simulink model "Shin_com"  (R2024a)
settings: Solver=VariableStepAuto  StartTime=0.0  StopTime=10.0  RelTol=1e-3
undefined symbols (not defined in the file): route1_waypoint_x, route1_waypoint_y, route2_waypoint_x, route2_waypoint_y, route3_waypoint_x, route3_waypoint_y, route4_waypoint_x, route4_waypoint_y, route5_waypoint_x, route5_waypoint_y
libraries: CarMaker4SL x162, slpidlib x4, robotalgslib x1, matrix_library x1
(part 2 of 4)

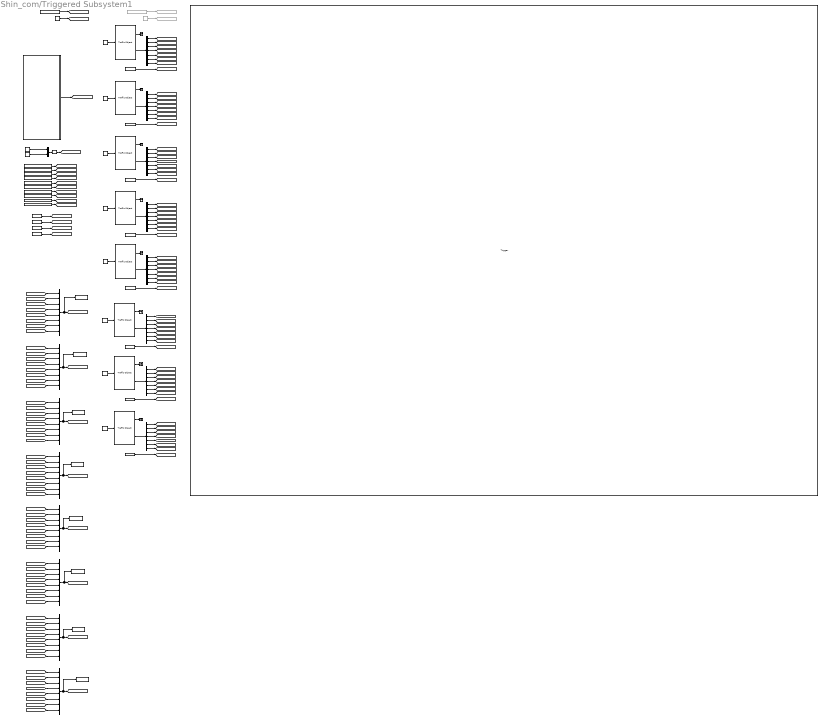
== system Shin_com/Triggered Subsystem1 ==
  note: Traffic Size
      | Length: 4.47
      | Width: 1.97
      | Height: 1.12
  note: Do Not Modify !!
  note: Traffic Size
      | Length: 4.47
      | Width: 1.97
      | Height: 1.12
  note: Traffic Size
      | Length: 4.47
      | Width: 1.97
      | Height: 1.12
  note: Traffic Size
      | Length: 4.47
      | Width: 1.97
      | Height: 1.12
  note: Do Not Modify !!
  note: Traffic Size
      | Length: 4.47
      | Width: 1.97
      | Height: 1.12
  note: Traffic Size
      | Length: 4.47
      | Width: 1.97
      | Height: 1.12
  note: Traffic Size
      | Length: 4.47
      | Width: 1.97
      | Height: 1.12
  note: Traffic Size
      | Length: 4.47
      | Width: 1.97
      | Height: 1.12
  Trigger : TriggerPort  TriggerType=function-call  VariantControl=(inherit)
      mask Display: image('KakaoTalk_20250521_163600732.jpg');
  Bus Selector{3..10} (8 alike) : BusSelector  OutputSignals=t_0 x,t_0 y,v_0 x,v_0 y,a_0 x,a_0 y,r_zyx z
  Constant11 : Constant  Value=28
  Constant12 : Constant  Value=route1_waypoint_y.Data
  Constant13 : Constant  Value=route2_waypoint_y.Data
  Constant14 : Constant  Value=route2_waypoint_x.Data
  Constant15 : Constant  Value=route1_waypoint_x.Data
  Constant16 : Constant  Value=route3_waypoint_y.Data
  Constant17 : Constant  Value=route3_waypoint_x.Data
  Constant18 : Constant  Value=route4_waypoint_y.Data
  Constant19 : Constant  Value=route4_waypoint_x.Data
  Constant20 : Constant  Value=route5_waypoint_y.Data
  Constant21 : Constant  Value=route5_waypoint_x.Data
  Constant22 : Constant  Value=23
  Constant23 : Constant  Value=10/3.6
  Constant25 : Constant  Value=11.5
  Constant26 : Constant  Value=24
  Constant27 : Constant  Value=25
  Constant28 : Constant  Value=26
  Constant29 : Constant  Value=27
  Constant6 : Constant  Commented=on  Value=20/3.6
  Constant7 : Constant  Value=21
  Constant8 : Constant  Value=2.48
  Constant9 : Constant  Value=22
  Goto31 : Goto  Commented=on  GotoTag=CrossTrackError
  Goto64 : Goto  Commented=on  GotoTag=Target_Speed
  Mux{,1..2,5..9} (8 alike) : Mux  Inputs=8
  Mux4 : Mux  Inputs=2
  Read CM Dict10 : CarMaker4SL/Read CM Dict  xname=Car.Fr1.tx  xsync=off  xstime=Inherited
  Read CM Dict11 : CarMaker4SL/Read CM Dict  xname=Car.Fr1.ty  xsync=off  xstime=Inherited
  Read CM Dict12 : CarMaker4SL/Read CM Dict  xname=Car.Fr1.rz  xsync=off  xstime=Inherited
  Read CM Dict13 : CarMaker4SL/Read CM Dict  xname=Car.v  xsync=off  xstime=Inherited
  Read CM Dict14 : CarMaker4SL/Read CM Dict  xname=Traffic.T24.rzv  xsync=off  xstime=Inherited
  Read CM Dict15 : CarMaker4SL/Read CM Dict  xname=Traffic.T25.rzv  xsync=off  xstime=Inherited
  Read CM Dict16 : CarMaker4SL/Read CM Dict  xname=Traffic.T26.rzv  xsync=off  xstime=Inherited
  Read CM Dict17 : CarMaker4SL/Read CM Dict  xname=Traffic.T27.rzv  xsync=off  xstime=Inherited
  Read CM Dict18 : CarMaker4SL/Read CM Dict  xname=Traffic.T28.rzv  xsync=off  xstime=Inherited
  Read CM Dict5 : CarMaker4SL/Read CM Dict  Commented=on  xname=Car.Road.Path.DevDist  xsync=off  xstime=Inherited
  Read CM Dict6 : CarMaker4SL/Read CM Dict  xname=Traffic.T21.rzv  xsync=off  xstime=Inherited
  Read CM Dict7 : CarMaker4SL/Read CM Dict  xname=Traffic.T22.rzv  xsync=off  xstime=Inherited
  Read CM Dict8 : CarMaker4SL/Read CM Dict  xname=Traffic.T23.rzv  xsync=off  xstime=Inherited
  Read CM Dict9 : CarMaker4SL/Read CM Dict  xname=Car.Road.Path.DevDist  xsync=off  xstime=Inherited
  Reshape2 : Reshape  OutputDimensionality=Row vector (2-D)  OutputDimensions=[2,2]
  Subsystem1 : Subsystem
  Terminator{3..9,11} (8 alike) : Terminator
  To Workspace : ToWorkspace  VariableName=obs_x  SaveFormat=Timeseries  SampleTime=-1
  To Workspace1 : ToWorkspace  VariableName=obs_Vx  SaveFormat=Timeseries  SampleTime=-1
  To Workspace2 : ToWorkspace  VariableName=obs_YawRate  SaveFormat=Timeseries  SampleTime=-1
  To Workspace3 : ToWorkspace  VariableName=obs_Ax  SaveFormat=Timeseries  SampleTime=-1
  To Workspace4 : ToWorkspace  VariableName=obs_y  SaveFormat=Timeseries  SampleTime=-1
  To Workspace5 : ToWorkspace  VariableName=obs_Vy  SaveFormat=Timeseries  SampleTime=-1
  To Workspace6 : ToWorkspace  VariableName=obs_Yaw  SaveFormat=Timeseries  SampleTime=-1
  To Workspace7 : ToWorkspace  VariableName=obs_Ay  SaveFormat=Timeseries  SampleTime=-1
  Traffic Object10 : CarMaker4SL/Traffic Object  xname=T28  ximode=Traffic Id  xstime=Inherited
      settings: SourceProductName=CarMaker4SL
  Traffic Object3 : CarMaker4SL/Traffic Object  xname=T21  ximode=Traffic Id  xstime=Inherited
      settings: SourceProductName=CarMaker4SL
  Traffic Object4 : CarMaker4SL/Traffic Object  xname=T22  ximode=Traffic Id  xstime=Inherited
      settings: SourceProductName=CarMaker4SL
  Traffic Object5 : CarMaker4SL/Traffic Object  xname=T23  ximode=Traffic Id  xstime=Inherited
      settings: SourceProductName=CarMaker4SL
  Traffic Object6 : CarMaker4SL/Traffic Object  xname=T24  ximode=Traffic Id  xstime=Inherited
      settings: SourceProductName=CarMaker4SL
  Traffic Object7 : CarMaker4SL/Traffic Object  xname=T25  ximode=Traffic Id  xstime=Inherited
      settings: SourceProductName=CarMaker4SL
  Traffic Object8 : CarMaker4SL/Traffic Object  xname=T26  ximode=Traffic Id  xstime=Inherited
      settings: SourceProductName=CarMaker4SL
  Traffic Object9 : CarMaker4SL/Traffic Object  xname=T27  ximode=Traffic Id  xstime=Inherited
      settings: SourceProductName=CarMaker4SL
  wires:
  [Traffic24_Ay] -> Mux9/4
  [Traffic26_Vy] -> Mux5/6
  [Traffic22_Global_Y] -> Mux1/2
  Bus Selector6/1 -> [Traffic24_Global_X]  "<t_0 x>"
  [Traffic26_YawRate] -> Mux6/6
  Read CM Dict14/1 -> [Traffic24_YawRate]
  [Traffic28_Ax] -> Mux8/8
  [Traffic21_Ax] -> Mux8/1
  [Traffic22_YawRate] -> Mux6/2
  Bus Selector6/2 -> [Traffic24_Global_Y]  "<t_0 y>"
  Bus Selector5/2 -> [Traffic23_Global_Y]  "<t_0 y>"
  Bus Selector6/7 -> [Traffic24_Yaw]  "<r_zyx z>"
  Constant29/1 -> Traffic Object9/1
  Read CM Dict5/1 -> Goto31/1
  [Traffic26_Ay] -> Mux9/6
  [Traffic22_Ax] -> Mux8/2
  Constant23/1 -> [Target_Speed]
  Bus Selector4/5 -> [Traffic22_Ax]  "<a_0 x>"
  Traffic Object7/1 -> Terminator7/1
  [Traffic21_Yaw] -> Mux7/1
  Bus Selector8/4 -> [Traffic26_Vy]  "<v_0 y>"
  [Traffic23_Vx] -> Mux2/3
  Bus Selector7/4 -> [Traffic25_Vy]  "<v_0 y>"
  Bus Selector3/3 -> [Traffic21_Vx]  "<v_0 x>"
  Reshape2/1 -> [Traffic_size]
  Constant12/1 -> [route1_waypoint_y]
  Bus Selector8/7 -> [Traffic26_Yaw]  "<r_zyx z>"
  Bus Selector9/4 -> [Traffic27_Vy]  "<v_0 y>"
  Read CM Dict12/1 -> [Ego_Yaw]
  Bus Selector9/2 -> [Traffic27_Global_Y]  "<t_0 y>"
  Mux6/1 -> To Workspace2/1, [obs_YawRate]
  Bus Selector8/6 -> [Traffic26_Ay]  "<a_0 y>"
  Constant13/1 -> [route2_waypoint_y]
  Constant11/1 -> Traffic Object10/1
  [Traffic22_Yaw] -> Mux7/2
  Mux7/1 -> To Workspace6/1, [obs_Yaw]
  [Traffic26_Ax] -> Mux8/6
  Bus Selector9/1 -> [Traffic27_Global_X]  "<t_0 x>"
  Traffic Object5/2 -> Bus Selector5/1
  Traffic Object6/2 -> Bus Selector6/1
  Bus Selector3/4 -> [Traffic21_Vy]  "<v_0 y>"
  Bus Selector10/7 -> [Traffic28_Yaw]  "<r_zyx z>"
  Bus Selector9/6 -> [Traffic27_Ay]  "<a_0 y>"
  [Traffic24_Global_Y] -> Mux1/4
  Bus Selector3/1 -> [Traffic21_Global_X]  "<t_0 x>"
  Read CM Dict13/1 -> [Ego_Vx]
  Constant14/1 -> [route2_waypoint_x]
  [Traffic28_Vx] -> Mux2/8
  Bus Selector6/5 -> [Traffic24_Ax]  "<a_0 x>"
  Bus Selector7/6 -> [Traffic25_Ay]  "<a_0 y>"
  Bus Selector8/3 -> [Traffic26_Vx]  "<v_0 x>"
  Constant15/1 -> [route1_waypoint_x]
  [Traffic27_Global_Y] -> Mux1/7
  Bus Selector10/4 -> [Traffic28_Vy]  "<v_0 y>"
  [Traffic23_YawRate] -> Mux6/3
  Bus Selector6/6 -> [Traffic24_Ay]  "<a_0 y>"
  [Traffic24_Ax] -> Mux8/4
  Bus Selector10/6 -> [Traffic28_Ay]  "<a_0 y>"
  [Traffic26_Vx] -> Mux2/6
  Read CM Dict17/1 -> [Traffic27_YawRate]
  [Traffic27_Ay] -> Mux9/7
  [Traffic26_Global_X] -> Mux/6
  Read CM Dict10/1 -> [Ego_Global_X]
  [Traffic27_YawRate] -> Mux6/7
  Mux5/1 -> To Workspace5/1, [obs_Vy]
  Bus Selector7/7 -> [Traffic25_Yaw]  "<r_zyx z>"
  Traffic Object8/2 -> Bus Selector8/1
  [Traffic28_Vx] -> Mux6/8
  [Traffic21_Ay] -> Mux9/1
  Mux2/1 -> To Workspace1/1, [obs_Vx]
  [Traffic21_Vx] -> Mux2/1
  [Traffic25_Vy] -> Mux5/5
  [Traffic23_Yaw] -> Mux7/3
  [Traffic28_Global_Y] -> Mux1/8
  [Traffic24_Yaw] -> Mux7/4
  Constant8/1 -> Mux4/1
  Bus Selector3/2 -> [Traffic21_Global_Y]  "<t_0 y>"
  [Traffic24_Vx] -> Mux2/4
  Read CM Dict11/1 -> [Ego_Gloabl_Y]
  Traffic Object6/1 -> Terminator6/1
  Read CM Dict16/1 -> [Traffic26_YawRate]
  Traffic Object4/2 -> Bus Selector4/1
  [Traffic25_YawRate] -> Mux6/5
  [Traffic23_Global_X] -> Mux/3
  Bus Selector10/5 -> [Traffic28_Ax]  "<a_0 x>"
  [Traffic28_Global_X] -> Mux/8
  Constant19/1 -> [route4_waypoint_x]
  [Traffic21_Global_X] -> Mux/1
  [Traffic24_YawRate] -> Mux6/4
  Traffic Object8/1 -> Terminator8/1
  [Traffic27_Vy] -> Mux5/7
  Bus Selector7/3 -> [Traffic25_Vx]  "<v_0 x>"
  Constant18/1 -> [route4_waypoint_y]
  [Traffic25_Vx] -> Mux2/5
  [Traffic21_Global_Y] -> Mux1/1
  Bus Selector5/4 -> [Traffic23_Vy]  "<v_0 y>"
  Constant21/1 -> [route5_waypoint_x]
  Read CM Dict7/1 -> [Traffic22_YawRate]
  Subsystem1/1(Traffic_Info) -> [Traffic_Info]
  Mux8/1 -> To Workspace3/1, [obs_Ax]
  Bus Selector8/2 -> [Traffic26_Global_Y]  "<t_0 y>"
  [Traffic26_Global_Y] -> Mux1/6
  Constant27/1 -> Traffic Object7/1
  [Traffic24_Global_X] -> Mux/4
  Constant9/1 -> Traffic Object4/1
  Bus Selector10/3 -> [Traffic28_Vx]  "<v_0 x>"
  [Traffic25_Yaw] -> Mux7/5
  [Traffic23_Ay] -> Mux9/3
  [Traffic22_Global_X] -> Mux/2
  Bus Selector10/1 -> [Traffic28_Global_X]  "<t_0 x>"
  Mux4/1 -> Reshape2/1
  Bus Selector5/5 -> [Traffic23_Ax]  "<a_0 x>"
  Bus Selector6/3 -> [Traffic24_Vx]  "<v_0 x>"
  Traffic Object3/1 -> Terminator3/1
  [Traffic23_Ax] -> Mux8/3
  Bus Selector10/2 -> [Traffic28_Global_Y]  "<t_0 y>"
  Mux1/1 -> To Workspace4/1, [obs_y]
  Bus Selector3/5 -> [Traffic21_Ax]  "<a_0 x>"
  [Traffic27_Global_X] -> Mux/7
  [Traffic25_Global_Y] -> Mux1/5
  Traffic Object4/1 -> Terminator4/1
  Constant7/1 -> Traffic Object3/1
  Read CM Dict18/1 -> [Traffic28_YawRate]
  Bus Selector9/5 -> [Traffic27_Ax]  "<a_0 x>"
  Bus Selector4/7 -> [Traffic22_Yaw]  "<r_zyx z>"
  [Traffic21_YawRate] -> Mux6/1
  Constant26/1 -> Traffic Object6/1
  Traffic Object7/2 -> Bus Selector7/1
  Bus Selector8/5 -> [Traffic26_Ax]  "<a_0 x>"
  [Traffic28_Ay] -> Mux9/8
  Read CM Dict9/1 -> [CrossTrackError]
  Read CM Dict8/1 -> [Traffic23_YawRate]
  Bus Selector7/1 -> [Traffic25_Global_X]  "<t_0 x>"
  [Traffic27_Vx] -> Mux2/7
  Traffic Object10/1 -> Terminator11/1
  Traffic Object9/2 -> Bus Selector9/1
  Constant16/1 -> [route3_waypoint_y]
  Constant22/1 -> Traffic Object5/1
  [Traffic21_Vy] -> Mux5/1
  Constant17/1 -> [route3_waypoint_x]
  Mux/1 -> To Workspace/1, [obs_x]
  Bus Selector7/2 -> [Traffic25_Global_Y]  "<t_0 y>"
  Bus Selector5/6 -> [Traffic23_Ay]  "<a_0 y>"
  [Traffic22_Vx] -> Mux2/2
  Constant6/1 -> Goto64/1
  [Traffic22_Vy] -> Mux5/2
  Bus Selector5/3 -> [Traffic23_Vx]  "<v_0 x>"
  Read CM Dict15/1 -> [Traffic25_YawRate]
  Traffic Object9/1 -> Terminator9/1
  Bus Selector9/7 -> [Traffic27_Yaw]  "<r_zyx z>"
  Bus Selector3/7 -> [Traffic21_Yaw]  "<r_zyx z>"
  [Traffic25_Ax] -> Mux8/5
  Read CM Dict6/1 -> [Traffic21_YawRate]
  Traffic Object3/2 -> Bus Selector3/1
  Bus Selector3/6 -> [Traffic21_Ay]  "<a_0 y>"
  Mux9/1 -> To Workspace7/1, [obs_Ay]
  Bus Selector8/1 -> [Traffic26_Global_X]  "<t_0 x>"
  [Traffic23_Vy] -> Mux5/3
  Constant28/1 -> Traffic Object8/1
  [Traffic23_Global_Y] -> Mux1/3
  [Traffic25_Ay] -> Mux9/5
  [Traffic26_Yaw] -> Mux7/6
  [Traffic22_Ay] -> Mux9/2
  Bus Selector4/3 -> [Traffic22_Vx]  "<v_0 x>"
  Constant20/1 -> [route5_waypoint_y]
  Bus Selector4/6 -> [Traffic22_Ay]  "<a_0 y>"
  [Traffic25_Global_X] -> Mux/5
  Bus Selector4/4 -> [Traffic22_Vy]  "<v_0 y>"
  [Traffic27_Ax] -> Mux8/7
  Traffic Object10/2 -> Bus Selector10/1
  Bus Selector9/3 -> [Traffic27_Vx]  "<v_0 x>"
  Bus Selector7/5 -> [Traffic25_Ax]  "<a_0 x>"
  [Traffic28_Yaw] -> Mux7/8
  Bus Selector5/7 -> [Traffic23_Yaw]  "<r_zyx z>"
  [Traffic24_Vy] -> Mux5/4
  Constant25/1 -> Mux4/2
  Bus Selector4/2 -> [Traffic22_Global_Y]  "<t_0 y>"
  Bus Selector5/1 -> [Traffic23_Global_X]  "<t_0 x>"
  [Traffic27_Yaw] -> Mux7/7
  [Traffic28_Vy] -> Mux5/8
  Bus Selector6/4 -> [Traffic24_Vy]  "<v_0 y>"
  Bus Selector4/1 -> [Traffic22_Global_X]  "<t_0 x>"
  Traffic Object5/1 -> Terminator5/1

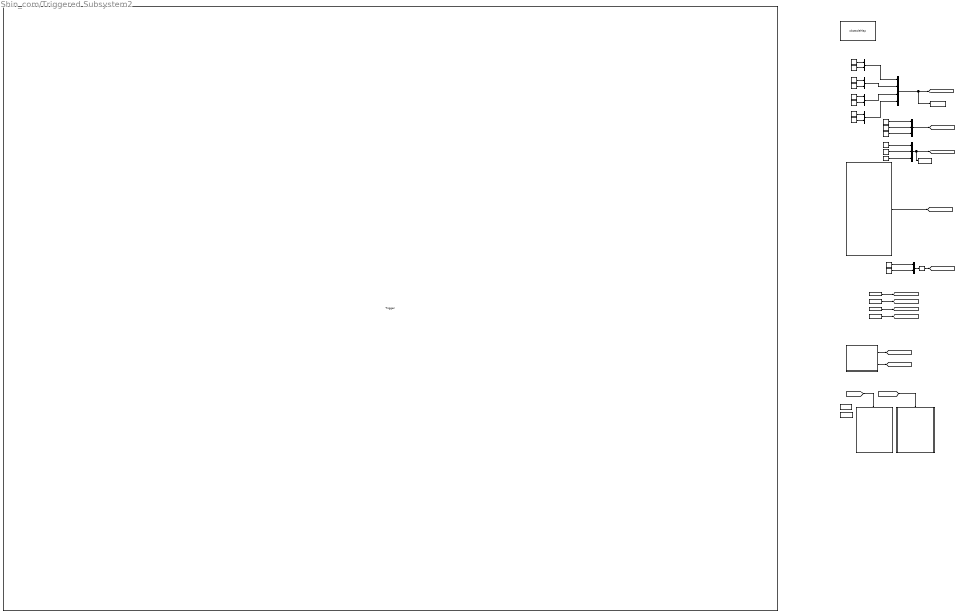
== system Shin_com/Triggered Subsystem2 ==
  note: Do Not Modify !!
  Trigger : TriggerPort  TriggerType=function-call  VariantControl=(inherit)
      mask Display: image('img.jpg');
  Chart1 : Stateflow chart  TreatAsAtomicUnit=on
      settings: PortSchema="{\"entries\":[{\"content\":{\"sides\":[{\"content\":{},\"type\":\"ConnectorPlacement.EquallySpacedRectSide\",\"uuid\":\"919f2d59-559a-485a-ad64-4ca203985945\"},{\"content\":{\"connectorIds\":[\"Out2\",\"Out1\"],\"side\":\"RIGHT\"},\"type\":\"ConnectorPlacement.EquallySpacedRectSide\",\"uuid\":\"5a15d665-f3e4-404a-9c46-468f267f06f6\"},{\"content\":{\"side\":\"TOP\"},\"type\":\"ConnectorPlacement.EquallySpacedRectSide\",\"uuid\":\"06264e3b-ed7f-4ae7-832b-fa30ed2f7930\"}]},\"type\":\"ConnectorPlacement.EquallySpacedConnector\",\"uuid\":\"55c66715-cf4a-4d9b-b78f-cac3e631d511\"}],\"packageUris\":[\"http://schema.mathworks.com/mf0/Connector/R2020b\"],\"version\":\"1.0\"}"
  Constant1 : Constant  Value=11.5
  Constant10 : Constant  Value=2.48
  Constant2 : Constant  Value=100
  Constant{5..6,24,32,36..37} (6 alike) : Constant  Value=0
  Constant3 : Constant  Value=-100
  Constant30 : Constant  Value=pi/2
  Constant33 : Constant  Value=-20
  Constant34 : Constant  Value=90
  Constant35 : Constant  Value=-3
  Constant38 : Constant  Value=-100
  Constant4 : Constant  Value=100
  Data Store Memory : DataStoreMemory  DataStoreName=obstacleMap  WriteAfterWriteMsg=warning  VectorParams1D=off  ShowAdditionalParam=off  Dimensions=[70 3]
  Data Store Memory1 : DataStoreMemory  DataStoreName=orderedPath  WriteAfterWriteMsg=warning  ShowAdditionalParam=off  Dimensions=[300 3]
  Data Store Memory2 : DataStoreMemory  DataStoreName=Finish_p  WriteAfterWriteMsg=warning  ShowAdditionalParam=off  Dimensions=[3 1]
  Data Store Write : DataStoreWrite  DataStoreName=Finish_p  IndexOptions=Index vector (dialog)  Indices=1  OutputSizes=1
  Function-Call Subsystem : Subsystem  TreatAsAtomicUnit=on
  Function-Call Subsystem1 : Subsystem  TreatAsAtomicUnit=on
  Mux10 : Mux  Inputs=3
  Mux{11..12,14..16} (5 alike) : Mux  Inputs=2
  Mux13 : Mux
  Mux3 : Mux  Inputs=3
  Read CM Dict1 : CarMaker4SL/Read CM Dict  xname=Car.Fr1.tx  xsync=off  xstime=Inherited
  Read CM Dict2 : CarMaker4SL/Read CM Dict  xname=Car.Fr1.ty  xsync=off  xstime=Inherited
  Read CM Dict3 : CarMaker4SL/Read CM Dict  xname=Car.Fr1.rz  xsync=off  xstime=Inherited
  Read CM Dict4 : CarMaker4SL/Read CM Dict  xname=Car.v  xsync=off  xstime=Inherited
  Reshape1 : Reshape  OutputDimensionality=Row vector (2-D)  OutputDimensions=[2,2]
  Subsystem : Subsystem
  To Workspace13 : ToWorkspace  VariableName=mapBoundary  SaveFormat=Timeseries  SampleTime=-1
  wires:
  Read CM Dict2/1 -> [Ego_Gloabl_Y]
  Constant2/1 -> Mux15/1
  Constant30/1 -> Mux10/3
  Read CM Dict1/1 -> [Ego_Global_X]
  Constant37/1 -> Mux11/2
  Mux10/1 -> [Finish_Point], Data Store Write/1
  Constant1/1 -> Mux12/2
  Mux11/1 -> Mux13/1
  Constant38/1 -> Mux14/2
  Mux3/1 -> [Start_Point]
  Mux13/1 -> [Map_Boundary], To Workspace13/1
  Constant35/1 -> Mux10/2
  Constant36/1 -> Mux14/1
  [go_Parking] -> Function-Call Subsystem1/Trigger
  Chart1/1(go_Parking()) -> [go_Parking]
  [draw_Map] -> Function-Call Subsystem/Trigger
  Constant10/1 -> Mux12/1
  Constant34/1 -> Mux10/1
  Constant5/1 -> Mux16/2
  Chart1/2(draw_Map()) -> [draw_Map]
  Mux16/1 -> Mux13/2
  Mux12/1 -> Reshape1/1
  Mux14/1 -> Mux13/4
  Constant33/1 -> Mux3/2
  Reshape1/1 -> [Traffic_size]
  Read CM Dict4/1 -> [Ego_Vx]
  Mux15/1 -> Mux13/3
  Read CM Dict3/1 -> [Ego_Yaw]
  Constant3/1 -> Mux15/2
  Constant32/1 -> Mux3/1
  Constant4/1 -> Mux16/1
  Constant24/1 -> Mux3/3
  Subsystem/1(Traffic_Info) -> [Traffic_Info]
  Constant6/1 -> Mux11/1

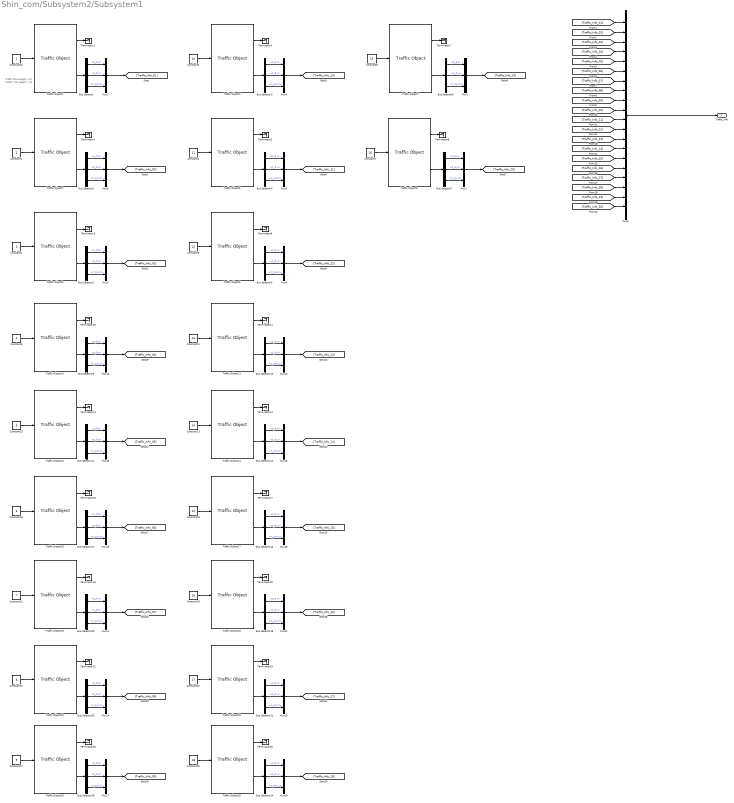
== system Shin_com/Subsystem2/Subsystem1 ==
  note: Traffic Size
      | Length: 4.47
      | Width: 1.97
      | Height: 1.12
  Bus Selector{,1..7,9..10,12,14..15,17..18,20..21,23..24,26} (20 alike) : BusSelector  OutputSignals=t_0 x,t_0 y,r_zyx z
  Constant1 : Constant  Value=2
  Constant10 : Constant
  Constant11 : Constant  Value=13
  Constant13 : Constant  Value=14
  Constant15 : Constant  Value=5
  Constant16 : Constant  Value=15
  Constant18 : Constant  Value=6
  Constant19 : Constant  Value=16
  Constant2 : Constant  Value=3
  Constant21 : Constant  Value=7
  Constant22 : Constant  Value=17
  Constant24 : Constant  Value=8
  Constant25 : Constant  Value=18
  Constant27 : Constant  Value=9
  Constant3 : Constant  Value=10
  Constant4 : Constant  Value=11
  Constant5 : Constant  Value=12
  Constant6 : Constant  Value=19
  Constant7 : Constant  Value=20
  Constant9 : Constant  Value=4
  Mux{1..8,12..13,15..16,18..19,21..22,24..25,27..28} (20 alike) : Mux  Inputs=3
  Mux9 : Mux  Inputs=20
  Terminator{1..8,10..11,13..14,16..17,19..20,22..23,25..26} (20 alike) : Terminator
  Traffic Object1 : CarMaker4SL/Traffic Object  xname=T01  ximode=Traffic Id  xstime=Inherited
      settings: SourceProductName=CarMaker4SL
  Traffic Object10 : CarMaker4SL/Traffic Object  xname=T04  ximode=Traffic Id  xstime=Inherited
      settings: SourceProductName=CarMaker4SL
  Traffic Object11 : CarMaker4SL/Traffic Object  xname=T13  ximode=Traffic Id  xstime=Inherited
      settings: SourceProductName=CarMaker4SL
  Traffic Object13 : CarMaker4SL/Traffic Object  xname=T05  ximode=Traffic Id  xstime=Inherited
      settings: SourceProductName=CarMaker4SL
  Traffic Object14 : CarMaker4SL/Traffic Object  xname=T14  ximode=Traffic Id  xstime=Inherited
      settings: SourceProductName=CarMaker4SL
  Traffic Object16 : CarMaker4SL/Traffic Object  xname=T06  ximode=Traffic Id  xstime=Inherited
      settings: SourceProductName=CarMaker4SL
  Traffic Object17 : CarMaker4SL/Traffic Object  xname=T15  ximode=Traffic Id  xstime=Inherited
      settings: SourceProductName=CarMaker4SL
  Traffic Object19 : CarMaker4SL/Traffic Object  xname=T07  ximode=Traffic Id  xstime=Inherited
      settings: SourceProductName=CarMaker4SL
  Traffic Object2 : CarMaker4SL/Traffic Object  xname=T02  ximode=Traffic Id  xstime=Inherited
      settings: SourceProductName=CarMaker4SL
  Traffic Object20 : CarMaker4SL/Traffic Object  xname=T16  ximode=Traffic Id  xstime=Inherited
      settings: SourceProductName=CarMaker4SL
  Traffic Object22 : CarMaker4SL/Traffic Object  xname=T08  ximode=Traffic Id  xstime=Inherited
      settings: SourceProductName=CarMaker4SL
  Traffic Object23 : CarMaker4SL/Traffic Object  xname=T17  ximode=Traffic Id  xstime=Inherited
      settings: SourceProductName=CarMaker4SL
  Traffic Object25 : CarMaker4SL/Traffic Object  xname=T03  ximode=Traffic Id  xstime=Inherited
      settings: SourceProductName=CarMaker4SL
  Traffic Object26 : CarMaker4SL/Traffic Object  xname=T18  ximode=Traffic Id  xstime=Inherited
      settings: SourceProductName=CarMaker4SL
  Traffic Object3 : CarMaker4SL/Traffic Object  xname=T03  ximode=Traffic Id  xstime=Inherited
      settings: SourceProductName=CarMaker4SL
  Traffic Object4 : CarMaker4SL/Traffic Object  xname=T10  ximode=Traffic Id  xstime=Inherited
      settings: SourceProductName=CarMaker4SL
  Traffic Object5 : CarMaker4SL/Traffic Object  xname=T11  ximode=Traffic Id  xstime=Inherited
      settings: SourceProductName=CarMaker4SL
  Traffic Object6 : CarMaker4SL/Traffic Object  xname=T12  ximode=Traffic Id  xstime=Inherited
      settings: SourceProductName=CarMaker4SL
  Traffic Object7 : CarMaker4SL/Traffic Object  xname=T19  ximode=Traffic Id  xstime=Inherited
      settings: SourceProductName=CarMaker4SL
  Traffic Object8 : CarMaker4SL/Traffic Object  xname=T20  ximode=Traffic Id  xstime=Inherited
      settings: SourceProductName=CarMaker4SL
  Traffic_Info : Outport
  wires:
  Constant10/1 -> Traffic Object1/1
  Traffic Object1/1 -> Terminator1/1
  Traffic Object2/1 -> Terminator2/1
  Constant1/1 -> Traffic Object2/1
  Constant2/1 -> Traffic Object3/1
  Traffic Object3/1 -> Terminator3/1
  Traffic Object4/1 -> Terminator4/1
  Constant3/1 -> Traffic Object4/1
  Constant4/1 -> Traffic Object5/1
  Traffic Object5/1 -> Terminator5/1
  Traffic Object6/1 -> Terminator6/1
  Constant5/1 -> Traffic Object6/1
  Constant6/1 -> Traffic Object7/1
  Traffic Object7/1 -> Terminator7/1
  Traffic Object1/2 -> Bus Selector/1
  Bus Selector/1 -> Mux2/1  "<t_0 x>"
  Bus Selector/2 -> Mux2/2  "<t_0 y>"
  Bus Selector/3 -> Mux2/3  "<r_zyx z>"
  Bus Selector1/2 -> Mux8/2  "<t_0 y>"
  Mux8/1 -> [Traffic_Info_02]
  Bus Selector1/1 -> Mux8/1  "<t_0 x>"
  Bus Selector1/3 -> Mux8/3  "<r_zyx z>"
  Traffic Object2/2 -> Bus Selector1/1
  Bus Selector2/2 -> Mux3/2  "<t_0 y>"
  Mux3/1 -> [Traffic_Info_03]
  Bus Selector2/1 -> Mux3/1  "<t_0 x>"
  Bus Selector2/3 -> Mux3/3  "<r_zyx z>"
  Traffic Object3/2 -> Bus Selector2/1
  Bus Selector3/2 -> Mux4/2  "<t_0 y>"
  Mux4/1 -> [Traffic_Info_10]
  Bus Selector3/1 -> Mux4/1  "<t_0 x>"
  Bus Selector3/3 -> Mux4/3  "<r_zyx z>"
  Traffic Object4/2 -> Bus Selector3/1
  Bus Selector4/2 -> Mux5/2  "<t_0 y>"
  Mux5/1 -> [Traffic_Info_11]
  Bus Selector4/1 -> Mux5/1  "<t_0 x>"
  Bus Selector4/3 -> Mux5/3  "<r_zyx z>"
  Traffic Object5/2 -> Bus Selector4/1
  Bus Selector5/2 -> Mux6/2  "<t_0 y>"
  Mux6/1 -> [Traffic_Info_12]
  Bus Selector5/1 -> Mux6/1  "<t_0 x>"
  Bus Selector5/3 -> Mux6/3  "<r_zyx z>"
  Traffic Object6/2 -> Bus Selector5/1
  Bus Selector6/2 -> Mux7/2  "<t_0 y>"
  Mux7/1 -> [Traffic_Info_19]
  Bus Selector6/1 -> Mux7/1  "<t_0 x>"
  Bus Selector6/3 -> Mux7/3  "<r_zyx z>"
  Traffic Object7/2 -> Bus Selector6/1
  Mux2/1 -> [Traffic_Info_01]
  Mux9/1 -> Traffic_Info/1
  Bus Selector7/3 -> Mux1/3  "<r_zyx z>"
  Traffic Object8/2 -> Bus Selector7/1
  Bus Selector7/2 -> Mux1/2  "<t_0 y>"
  Mux1/1 -> [Traffic_Info_20]
  Traffic Object8/1 -> Terminator8/1
  Constant7/1 -> Traffic Object8/1
  Bus Selector7/1 -> Mux1/1  "<t_0 x>"
  Bus Selector10/3 -> Mux13/3  "<r_zyx z>"
  Traffic Object10/2 -> Bus Selector9/1
  Constant11/1 -> Traffic Object11/1
  Bus Selector10/1 -> Mux13/1  "<t_0 x>"
  Traffic Object11/2 -> Bus Selector10/1
  Mux13/1 -> [Traffic_Info_13]
  Bus Selector10/2 -> Mux13/2  "<t_0 y>"
  Mux12/1 -> [Traffic_Info_04]
  Bus Selector9/2 -> Mux12/2  "<t_0 y>"
  Traffic Object11/1 -> Terminator11/1
  Bus Selector9/1 -> Mux12/1  "<t_0 x>"
  Constant9/1 -> Traffic Object10/1
  Traffic Object10/1 -> Terminator10/1
  Bus Selector9/3 -> Mux12/3  "<r_zyx z>"
  Bus Selector14/2 -> Mux15/2  "<t_0 y>"
  Mux15/1 -> [Traffic_Info_05]
  Mux16/1 -> [Traffic_Info_14]
  Traffic Object14/1 -> Terminator14/1
  Bus Selector12/2 -> Mux16/2  "<t_0 y>"
  Traffic Object14/2 -> Bus Selector12/1
  Bus Selector12/1 -> Mux16/1  "<t_0 x>"
  Constant13/1 -> Traffic Object14/1
  Bus Selector12/3 -> Mux16/3  "<r_zyx z>"
  Traffic Object13/2 -> Bus Selector14/1
  Bus Selector14/1 -> Mux15/1  "<t_0 x>"
  Bus Selector14/3 -> Mux15/3  "<r_zyx z>"
  Traffic Object13/1 -> Terminator13/1
  Constant15/1 -> Traffic Object13/1
  Bus Selector17/2 -> Mux18/2  "<t_0 y>"
  Mux18/1 -> [Traffic_Info_06]
  Mux19/1 -> [Traffic_Info_15]
  Traffic Object17/1 -> Terminator17/1
  Bus Selector15/2 -> Mux19/2  "<t_0 y>"
  Traffic Object17/2 -> Bus Selector15/1
  Bus Selector15/1 -> Mux19/1  "<t_0 x>"
  Constant16/1 -> Traffic Object17/1
  Bus Selector15/3 -> Mux19/3  "<r_zyx z>"
  Traffic Object16/2 -> Bus Selector17/1
  Bus Selector17/1 -> Mux18/1  "<t_0 x>"
  Bus Selector17/3 -> Mux18/3  "<r_zyx z>"
  Traffic Object16/1 -> Terminator16/1
  Constant18/1 -> Traffic Object16/1
  Bus Selector20/2 -> Mux21/2  "<t_0 y>"
  Mux21/1 -> [Traffic_Info_07]
  Mux22/1 -> [Traffic_Info_16]
  Traffic Object20/1 -> Terminator20/1
  Bus Selector18/2 -> Mux22/2  "<t_0 y>"
  Traffic Object20/2 -> Bus Selector18/1
  Bus Selector18/1 -> Mux22/1  "<t_0 x>"
  Constant19/1 -> Traffic Object20/1
  Bus Selector18/3 -> Mux22/3  "<r_zyx z>"
  Traffic Object19/2 -> Bus Selector20/1
  Bus Selector20/1 -> Mux21/1  "<t_0 x>"
  Bus Selector20/3 -> Mux21/3  "<r_zyx z>"
  Traffic Object19/1 -> Terminator19/1
  Constant21/1 -> Traffic Object19/1
  Bus Selector23/2 -> Mux24/2  "<t_0 y>"
  Mux24/1 -> [Traffic_Info_08]
  Mux25/1 -> [Traffic_Info_17]
  Traffic Object23/1 -> Terminator23/1
  Bus Selector21/2 -> Mux25/2  "<t_0 y>"
  Traffic Object23/2 -> Bus Selector21/1
  Bus Selector21/1 -> Mux25/1  "<t_0 x>"
  Constant22/1 -> Traffic Object23/1
  Bus Selector21/3 -> Mux25/3  "<r_zyx z>"
  Traffic Object22/2 -> Bus Selector23/1
  Bus Selector23/1 -> Mux24/1  "<t_0 x>"
  Bus Selector23/3 -> Mux24/3  "<r_zyx z>"
  Traffic Object22/1 -> Terminator22/1
  Constant24/1 -> Traffic Object22/1
  Bus Selector26/2 -> Mux27/2  "<t_0 y>"
  Mux27/1 -> [Traffic_Info_09]
  Mux28/1 -> [Traffic_Info_18]
  Traffic Object26/1 -> Terminator26/1
  Bus Selector24/2 -> Mux28/2  "<t_0 y>"
  Traffic Object26/2 -> Bus Selector24/1
  Bus Selector24/1 -> Mux28/1  "<t_0 x>"
  Constant25/1 -> Traffic Object26/1
  Bus Selector24/3 -> Mux28/3  "<r_zyx z>"
  Traffic Object25/2 -> Bus Selector26/1
  Bus Selector26/1 -> Mux27/1  "<t_0 x>"
  Bus Selector26/3 -> Mux27/3  "<r_zyx z>"
  Traffic Object25/1 -> Terminator25/1
  Constant27/1 -> Traffic Object25/1
  [Traffic_Info_01] -> Mux9/1
  [Traffic_Info_02] -> Mux9/2
  [Traffic_Info_03] -> Mux9/3
  [Traffic_Info_04] -> Mux9/4
  [Traffic_Info_05] -> Mux9/5
  [Traffic_Info_06] -> Mux9/6
  [Traffic_Info_07] -> Mux9/7
  [Traffic_Info_08] -> Mux9/8
  [Traffic_Info_09] -> Mux9/9
  [Traffic_Info_10] -> Mux9/10
  [Traffic_Info_11] -> Mux9/11
  [Traffic_Info_12] -> Mux9/12
  [Traffic_Info_13] -> Mux9/13
  [Traffic_Info_14] -> Mux9/14
  [Traffic_Info_15] -> Mux9/15
  [Traffic_Info_16] -> Mux9/16
  [Traffic_Info_17] -> Mux9/17
  [Traffic_Info_18] -> Mux9/18
  [Traffic_Info_19] -> Mux9/19
  [Traffic_Info_20] -> Mux9/20

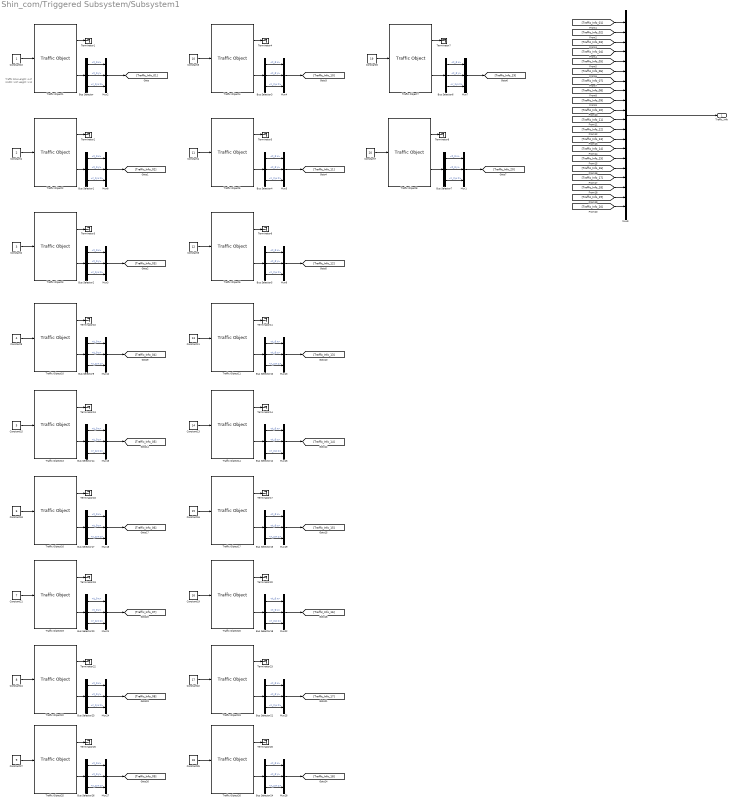
== system Shin_com/Triggered Subsystem/Subsystem1 ==
  note: Traffic Size
      | Length: 4.47
      | Width: 1.97
      | Height: 1.12
  Bus Selector{,1..7,9..10,12,14..15,17..18,20..21,23..24,26} (20 alike) : BusSelector  OutputSignals=t_0 x,t_0 y,r_zyx z
  Constant1 : Constant  Value=2
  Constant10 : Constant
  Constant11 : Constant  Value=13
  Constant13 : Constant  Value=14
  Constant15 : Constant  Value=5
  Constant16 : Constant  Value=15
  Constant18 : Constant  Value=6
  Constant19 : Constant  Value=16
  Constant2 : Constant  Value=3
  Constant21 : Constant  Value=7
  Constant22 : Constant  Value=17
  Constant24 : Constant  Value=8
  Constant25 : Constant  Value=18
  Constant27 : Constant  Value=9
  Constant3 : Constant  Value=10
  Constant4 : Constant  Value=11
  Constant5 : Constant  Value=12
  Constant6 : Constant  Value=19
  Constant7 : Constant  Value=20
  Constant9 : Constant  Value=4
  Mux{1..8,12..13,15..16,18..19,21..22,24..25,27..28} (20 alike) : Mux  Inputs=3
  Mux9 : Mux  Inputs=20
  Terminator{1..8,10..11,13..14,16..17,19..20,22..23,25..26} (20 alike) : Terminator
  Traffic Object1 : CarMaker4SL/Traffic Object  xname=T01  ximode=Traffic Id  xstime=Inherited
      settings: SourceProductName=CarMaker4SL
  Traffic Object10 : CarMaker4SL/Traffic Object  xname=T04  ximode=Traffic Id  xstime=Inherited
      settings: SourceProductName=CarMaker4SL
  Traffic Object11 : CarMaker4SL/Traffic Object  xname=T13  ximode=Traffic Id  xstime=Inherited
      settings: SourceProductName=CarMaker4SL
  Traffic Object13 : CarMaker4SL/Traffic Object  xname=T05  ximode=Traffic Id  xstime=Inherited
      settings: SourceProductName=CarMaker4SL
  Traffic Object14 : CarMaker4SL/Traffic Object  xname=T14  ximode=Traffic Id  xstime=Inherited
      settings: SourceProductName=CarMaker4SL
  Traffic Object16 : CarMaker4SL/Traffic Object  xname=T06  ximode=Traffic Id  xstime=Inherited
      settings: SourceProductName=CarMaker4SL
  Traffic Object17 : CarMaker4SL/Traffic Object  xname=T15  ximode=Traffic Id  xstime=Inherited
      settings: SourceProductName=CarMaker4SL
  Traffic Object19 : CarMaker4SL/Traffic Object  xname=T07  ximode=Traffic Id  xstime=Inherited
      settings: SourceProductName=CarMaker4SL
  Traffic Object2 : CarMaker4SL/Traffic Object  xname=T02  ximode=Traffic Id  xstime=Inherited
      settings: SourceProductName=CarMaker4SL
  Traffic Object20 : CarMaker4SL/Traffic Object  xname=T16  ximode=Traffic Id  xstime=Inherited
      settings: SourceProductName=CarMaker4SL
  Traffic Object22 : CarMaker4SL/Traffic Object  xname=T08  ximode=Traffic Id  xstime=Inherited
      settings: SourceProductName=CarMaker4SL
  Traffic Object23 : CarMaker4SL/Traffic Object  xname=T17  ximode=Traffic Id  xstime=Inherited
      settings: SourceProductName=CarMaker4SL
  Traffic Object25 : CarMaker4SL/Traffic Object  xname=T03  ximode=Traffic Id  xstime=Inherited
      settings: SourceProductName=CarMaker4SL
  Traffic Object26 : CarMaker4SL/Traffic Object  xname=T18  ximode=Traffic Id  xstime=Inherited
      settings: SourceProductName=CarMaker4SL
  Traffic Object3 : CarMaker4SL/Traffic Object  xname=T03  ximode=Traffic Id  xstime=Inherited
      settings: SourceProductName=CarMaker4SL
  Traffic Object4 : CarMaker4SL/Traffic Object  xname=T10  ximode=Traffic Id  xstime=Inherited
      settings: SourceProductName=CarMaker4SL
  Traffic Object5 : CarMaker4SL/Traffic Object  xname=T11  ximode=Traffic Id  xstime=Inherited
      settings: SourceProductName=CarMaker4SL
  Traffic Object6 : CarMaker4SL/Traffic Object  xname=T12  ximode=Traffic Id  xstime=Inherited
      settings: SourceProductName=CarMaker4SL
  Traffic Object7 : CarMaker4SL/Traffic Object  xname=T19  ximode=Traffic Id  xstime=Inherited
      settings: SourceProductName=CarMaker4SL
  Traffic Object8 : CarMaker4SL/Traffic Object  xname=T20  ximode=Traffic Id  xstime=Inherited
      settings: SourceProductName=CarMaker4SL
  Traffic_Info : Outport
  wires:
  Constant10/1 -> Traffic Object1/1
  Traffic Object1/1 -> Terminator1/1
  Traffic Object2/1 -> Terminator2/1
  Constant1/1 -> Traffic Object2/1
  Constant2/1 -> Traffic Object3/1
  Traffic Object3/1 -> Terminator3/1
  Traffic Object4/1 -> Terminator4/1
  Constant3/1 -> Traffic Object4/1
  Constant4/1 -> Traffic Object5/1
  Traffic Object5/1 -> Terminator5/1
  Traffic Object6/1 -> Terminator6/1
  Constant5/1 -> Traffic Object6/1
  Constant6/1 -> Traffic Object7/1
  Traffic Object7/1 -> Terminator7/1
  Traffic Object1/2 -> Bus Selector/1
  Bus Selector/1 -> Mux2/1  "<t_0 x>"
  Bus Selector/2 -> Mux2/2  "<t_0 y>"
  Bus Selector/3 -> Mux2/3  "<r_zyx z>"
  Bus Selector1/2 -> Mux8/2  "<t_0 y>"
  Mux8/1 -> [Traffic_Info_02]
  Bus Selector1/1 -> Mux8/1  "<t_0 x>"
  Bus Selector1/3 -> Mux8/3  "<r_zyx z>"
  Traffic Object2/2 -> Bus Selector1/1
  Bus Selector2/2 -> Mux3/2  "<t_0 y>"
  Mux3/1 -> [Traffic_Info_03]
  Bus Selector2/1 -> Mux3/1  "<t_0 x>"
  Bus Selector2/3 -> Mux3/3  "<r_zyx z>"
  Traffic Object3/2 -> Bus Selector2/1
  Bus Selector3/2 -> Mux4/2  "<t_0 y>"
  Mux4/1 -> [Traffic_Info_10]
  Bus Selector3/1 -> Mux4/1  "<t_0 x>"
  Bus Selector3/3 -> Mux4/3  "<r_zyx z>"
  Traffic Object4/2 -> Bus Selector3/1
  Bus Selector4/2 -> Mux5/2  "<t_0 y>"
  Mux5/1 -> [Traffic_Info_11]
  Bus Selector4/1 -> Mux5/1  "<t_0 x>"
  Bus Selector4/3 -> Mux5/3  "<r_zyx z>"
  Traffic Object5/2 -> Bus Selector4/1
  Bus Selector5/2 -> Mux6/2  "<t_0 y>"
  Mux6/1 -> [Traffic_Info_12]
  Bus Selector5/1 -> Mux6/1  "<t_0 x>"
  Bus Selector5/3 -> Mux6/3  "<r_zyx z>"
  Traffic Object6/2 -> Bus Selector5/1
  Bus Selector6/2 -> Mux7/2  "<t_0 y>"
  Mux7/1 -> [Traffic_Info_19]
  Bus Selector6/1 -> Mux7/1  "<t_0 x>"
  Bus Selector6/3 -> Mux7/3  "<r_zyx z>"
  Traffic Object7/2 -> Bus Selector6/1
  Mux2/1 -> [Traffic_Info_01]
  Mux9/1 -> Traffic_Info/1
  Bus Selector7/3 -> Mux1/3  "<r_zyx z>"
  Traffic Object8/2 -> Bus Selector7/1
  Bus Selector7/2 -> Mux1/2  "<t_0 y>"
  Mux1/1 -> [Traffic_Info_20]
  Traffic Object8/1 -> Terminator8/1
  Constant7/1 -> Traffic Object8/1
  Bus Selector7/1 -> Mux1/1  "<t_0 x>"
  Bus Selector10/3 -> Mux13/3  "<r_zyx z>"
  Traffic Object10/2 -> Bus Selector9/1
  Constant11/1 -> Traffic Object11/1
  Bus Selector10/1 -> Mux13/1  "<t_0 x>"
  Traffic Object11/2 -> Bus Selector10/1
  Mux13/1 -> [Traffic_Info_13]
  Bus Selector10/2 -> Mux13/2  "<t_0 y>"
  Mux12/1 -> [Traffic_Info_04]
  Bus Selector9/2 -> Mux12/2  "<t_0 y>"
  Traffic Object11/1 -> Terminator11/1
  Bus Selector9/1 -> Mux12/1  "<t_0 x>"
  Constant9/1 -> Traffic Object10/1
  Traffic Object10/1 -> Terminator10/1
  Bus Selector9/3 -> Mux12/3  "<r_zyx z>"
  Bus Selector14/2 -> Mux15/2  "<t_0 y>"
  Mux15/1 -> [Traffic_Info_05]
  Mux16/1 -> [Traffic_Info_14]
  Traffic Object14/1 -> Terminator14/1
  Bus Selector12/2 -> Mux16/2  "<t_0 y>"
  Traffic Object14/2 -> Bus Selector12/1
  Bus Selector12/1 -> Mux16/1  "<t_0 x>"
  Constant13/1 -> Traffic Object14/1
  Bus Selector12/3 -> Mux16/3  "<r_zyx z>"
  Traffic Object13/2 -> Bus Selector14/1
  Bus Selector14/1 -> Mux15/1  "<t_0 x>"
  Bus Selector14/3 -> Mux15/3  "<r_zyx z>"
  Traffic Object13/1 -> Terminator13/1
  Constant15/1 -> Traffic Object13/1
  Bus Selector17/2 -> Mux18/2  "<t_0 y>"
  Mux18/1 -> [Traffic_Info_06]
  Mux19/1 -> [Traffic_Info_15]
  Traffic Object17/1 -> Terminator17/1
  Bus Selector15/2 -> Mux19/2  "<t_0 y>"
  Traffic Object17/2 -> Bus Selector15/1
  Bus Selector15/1 -> Mux19/1  "<t_0 x>"
  Constant16/1 -> Traffic Object17/1
  Bus Selector15/3 -> Mux19/3  "<r_zyx z>"
  Traffic Object16/2 -> Bus Selector17/1
  Bus Selector17/1 -> Mux18/1  "<t_0 x>"
  Bus Selector17/3 -> Mux18/3  "<r_zyx z>"
  Traffic Object16/1 -> Terminator16/1
  Constant18/1 -> Traffic Object16/1
  Bus Selector20/2 -> Mux21/2  "<t_0 y>"
  Mux21/1 -> [Traffic_Info_07]
  Mux22/1 -> [Traffic_Info_16]
  Traffic Object20/1 -> Terminator20/1
  Bus Selector18/2 -> Mux22/2  "<t_0 y>"
  Traffic Object20/2 -> Bus Selector18/1
  Bus Selector18/1 -> Mux22/1  "<t_0 x>"
  Constant19/1 -> Traffic Object20/1
  Bus Selector18/3 -> Mux22/3  "<r_zyx z>"
  Traffic Object19/2 -> Bus Selector20/1
  Bus Selector20/1 -> Mux21/1  "<t_0 x>"
  Bus Selector20/3 -> Mux21/3  "<r_zyx z>"
  Traffic Object19/1 -> Terminator19/1
  Constant21/1 -> Traffic Object19/1
  Bus Selector23/2 -> Mux24/2  "<t_0 y>"
  Mux24/1 -> [Traffic_Info_08]
  Mux25/1 -> [Traffic_Info_17]
  Traffic Object23/1 -> Terminator23/1
  Bus Selector21/2 -> Mux25/2  "<t_0 y>"
  Traffic Object23/2 -> Bus Selector21/1
  Bus Selector21/1 -> Mux25/1  "<t_0 x>"
  Constant22/1 -> Traffic Object23/1
  Bus Selector21/3 -> Mux25/3  "<r_zyx z>"
  Traffic Object22/2 -> Bus Selector23/1
  Bus Selector23/1 -> Mux24/1  "<t_0 x>"
  Bus Selector23/3 -> Mux24/3  "<r_zyx z>"
  Traffic Object22/1 -> Terminator22/1
  Constant24/1 -> Traffic Object22/1
  Bus Selector26/2 -> Mux27/2  "<t_0 y>"
  Mux27/1 -> [Traffic_Info_09]
  Mux28/1 -> [Traffic_Info_18]
  Traffic Object26/1 -> Terminator26/1
  Bus Selector24/2 -> Mux28/2  "<t_0 y>"
  Traffic Object26/2 -> Bus Selector24/1
  Bus Selector24/1 -> Mux28/1  "<t_0 x>"
  Constant25/1 -> Traffic Object26/1
  Bus Selector24/3 -> Mux28/3  "<r_zyx z>"
  Traffic Object25/2 -> Bus Selector26/1
  Bus Selector26/1 -> Mux27/1  "<t_0 x>"
  Bus Selector26/3 -> Mux27/3  "<r_zyx z>"
  Traffic Object25/1 -> Terminator25/1
  Constant27/1 -> Traffic Object25/1
  [Traffic_Info_01] -> Mux9/1
  [Traffic_Info_02] -> Mux9/2
  [Traffic_Info_03] -> Mux9/3
  [Traffic_Info_04] -> Mux9/4
  [Traffic_Info_05] -> Mux9/5
  [Traffic_Info_06] -> Mux9/6
  [Traffic_Info_07] -> Mux9/7
  [Traffic_Info_08] -> Mux9/8
  [Traffic_Info_09] -> Mux9/9
  [Traffic_Info_10] -> Mux9/10
  [Traffic_Info_11] -> Mux9/11
  [Traffic_Info_12] -> Mux9/12
  [Traffic_Info_13] -> Mux9/13
  [Traffic_Info_14] -> Mux9/14
  [Traffic_Info_15] -> Mux9/15
  [Traffic_Info_16] -> Mux9/16
  [Traffic_Info_17] -> Mux9/17
  [Traffic_Info_18] -> Mux9/18
  [Traffic_Info_19] -> Mux9/19
  [Traffic_Info_20] -> Mux9/20

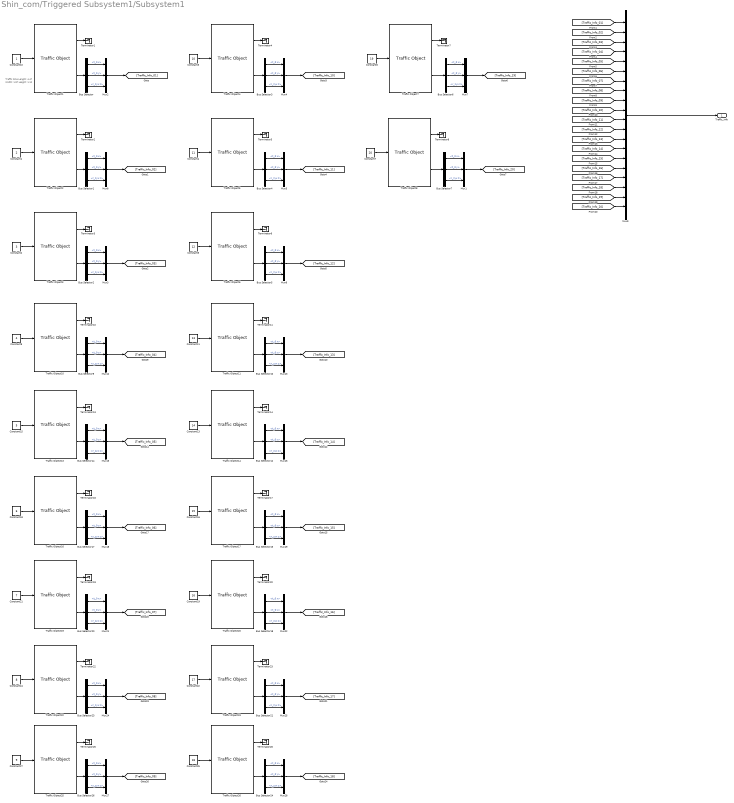
== system Shin_com/Triggered Subsystem1/Subsystem1 ==
  note: Traffic Size
      | Length: 4.47
      | Width: 1.97
      | Height: 1.12
  Bus Selector{,1..7,9..10,12,14..15,17..18,20..21,23..24,26} (20 alike) : BusSelector  OutputSignals=t_0 x,t_0 y,r_zyx z
  Constant1 : Constant  Value=2
  Constant10 : Constant
  Constant11 : Constant  Value=13
  Constant13 : Constant  Value=14
  Constant15 : Constant  Value=5
  Constant16 : Constant  Value=15
  Constant18 : Constant  Value=6
  Constant19 : Constant  Value=16
  Constant2 : Constant  Value=3
  Constant21 : Constant  Value=7
  Constant22 : Constant  Value=17
  Constant24 : Constant  Value=8
  Constant25 : Constant  Value=18
  Constant27 : Constant  Value=9
  Constant3 : Constant  Value=10
  Constant4 : Constant  Value=11
  Constant5 : Constant  Value=12
  Constant6 : Constant  Value=19
  Constant7 : Constant  Value=20
  Constant9 : Constant  Value=4
  Mux{1..8,12..13,15..16,18..19,21..22,24..25,27..28} (20 alike) : Mux  Inputs=3
  Mux9 : Mux  Inputs=20
  Terminator{1..8,10..11,13..14,16..17,19..20,22..23,25..26} (20 alike) : Terminator
  Traffic Object1 : CarMaker4SL/Traffic Object  xname=T01  ximode=Traffic Id  xstime=Inherited
      settings: SourceProductName=CarMaker4SL
  Traffic Object10 : CarMaker4SL/Traffic Object  xname=T04  ximode=Traffic Id  xstime=Inherited
      settings: SourceProductName=CarMaker4SL
  Traffic Object11 : CarMaker4SL/Traffic Object  xname=T13  ximode=Traffic Id  xstime=Inherited
      settings: SourceProductName=CarMaker4SL
  Traffic Object13 : CarMaker4SL/Traffic Object  xname=T05  ximode=Traffic Id  xstime=Inherited
      settings: SourceProductName=CarMaker4SL
  Traffic Object14 : CarMaker4SL/Traffic Object  xname=T14  ximode=Traffic Id  xstime=Inherited
      settings: SourceProductName=CarMaker4SL
  Traffic Object16 : CarMaker4SL/Traffic Object  xname=T06  ximode=Traffic Id  xstime=Inherited
      settings: SourceProductName=CarMaker4SL
  Traffic Object17 : CarMaker4SL/Traffic Object  xname=T15  ximode=Traffic Id  xstime=Inherited
      settings: SourceProductName=CarMaker4SL
  Traffic Object19 : CarMaker4SL/Traffic Object  xname=T07  ximode=Traffic Id  xstime=Inherited
      settings: SourceProductName=CarMaker4SL
  Traffic Object2 : CarMaker4SL/Traffic Object  xname=T02  ximode=Traffic Id  xstime=Inherited
      settings: SourceProductName=CarMaker4SL
  Traffic Object20 : CarMaker4SL/Traffic Object  xname=T16  ximode=Traffic Id  xstime=Inherited
      settings: SourceProductName=CarMaker4SL
  Traffic Object22 : CarMaker4SL/Traffic Object  xname=T08  ximode=Traffic Id  xstime=Inherited
      settings: SourceProductName=CarMaker4SL
  Traffic Object23 : CarMaker4SL/Traffic Object  xname=T17  ximode=Traffic Id  xstime=Inherited
      settings: SourceProductName=CarMaker4SL
  Traffic Object25 : CarMaker4SL/Traffic Object  xname=T03  ximode=Traffic Id  xstime=Inherited
      settings: SourceProductName=CarMaker4SL
  Traffic Object26 : CarMaker4SL/Traffic Object  xname=T18  ximode=Traffic Id  xstime=Inherited
      settings: SourceProductName=CarMaker4SL
  Traffic Object3 : CarMaker4SL/Traffic Object  xname=T03  ximode=Traffic Id  xstime=Inherited
      settings: SourceProductName=CarMaker4SL
  Traffic Object4 : CarMaker4SL/Traffic Object  xname=T10  ximode=Traffic Id  xstime=Inherited
      settings: SourceProductName=CarMaker4SL
  Traffic Object5 : CarMaker4SL/Traffic Object  xname=T11  ximode=Traffic Id  xstime=Inherited
      settings: SourceProductName=CarMaker4SL
  Traffic Object6 : CarMaker4SL/Traffic Object  xname=T12  ximode=Traffic Id  xstime=Inherited
      settings: SourceProductName=CarMaker4SL
  Traffic Object7 : CarMaker4SL/Traffic Object  xname=T19  ximode=Traffic Id  xstime=Inherited
      settings: SourceProductName=CarMaker4SL
  Traffic Object8 : CarMaker4SL/Traffic Object  xname=T20  ximode=Traffic Id  xstime=Inherited
      settings: SourceProductName=CarMaker4SL
  Traffic_Info : Outport
  wires:
  Constant10/1 -> Traffic Object1/1
  Traffic Object1/1 -> Terminator1/1
  Traffic Object2/1 -> Terminator2/1
  Constant1/1 -> Traffic Object2/1
  Constant2/1 -> Traffic Object3/1
  Traffic Object3/1 -> Terminator3/1
  Traffic Object4/1 -> Terminator4/1
  Constant3/1 -> Traffic Object4/1
  Constant4/1 -> Traffic Object5/1
  Traffic Object5/1 -> Terminator5/1
  Traffic Object6/1 -> Terminator6/1
  Constant5/1 -> Traffic Object6/1
  Constant6/1 -> Traffic Object7/1
  Traffic Object7/1 -> Terminator7/1
  Traffic Object1/2 -> Bus Selector/1
  Bus Selector/1 -> Mux2/1  "<t_0 x>"
  Bus Selector/2 -> Mux2/2  "<t_0 y>"
  Bus Selector/3 -> Mux2/3  "<r_zyx z>"
  Bus Selector1/2 -> Mux8/2  "<t_0 y>"
  Mux8/1 -> [Traffic_Info_02]
  Bus Selector1/1 -> Mux8/1  "<t_0 x>"
  Bus Selector1/3 -> Mux8/3  "<r_zyx z>"
  Traffic Object2/2 -> Bus Selector1/1
  Bus Selector2/2 -> Mux3/2  "<t_0 y>"
  Mux3/1 -> [Traffic_Info_03]
  Bus Selector2/1 -> Mux3/1  "<t_0 x>"
  Bus Selector2/3 -> Mux3/3  "<r_zyx z>"
  Traffic Object3/2 -> Bus Selector2/1
  Bus Selector3/2 -> Mux4/2  "<t_0 y>"
  Mux4/1 -> [Traffic_Info_10]
  Bus Selector3/1 -> Mux4/1  "<t_0 x>"
  Bus Selector3/3 -> Mux4/3  "<r_zyx z>"
  Traffic Object4/2 -> Bus Selector3/1
  Bus Selector4/2 -> Mux5/2  "<t_0 y>"
  Mux5/1 -> [Traffic_Info_11]
  Bus Selector4/1 -> Mux5/1  "<t_0 x>"
  Bus Selector4/3 -> Mux5/3  "<r_zyx z>"
  Traffic Object5/2 -> Bus Selector4/1
  Bus Selector5/2 -> Mux6/2  "<t_0 y>"
  Mux6/1 -> [Traffic_Info_12]
  Bus Selector5/1 -> Mux6/1  "<t_0 x>"
  Bus Selector5/3 -> Mux6/3  "<r_zyx z>"
  Traffic Object6/2 -> Bus Selector5/1
  Bus Selector6/2 -> Mux7/2  "<t_0 y>"
  Mux7/1 -> [Traffic_Info_19]
  Bus Selector6/1 -> Mux7/1  "<t_0 x>"
  Bus Selector6/3 -> Mux7/3  "<r_zyx z>"
  Traffic Object7/2 -> Bus Selector6/1
  Mux2/1 -> [Traffic_Info_01]
  Mux9/1 -> Traffic_Info/1
  Bus Selector7/3 -> Mux1/3  "<r_zyx z>"
  Traffic Object8/2 -> Bus Selector7/1
  Bus Selector7/2 -> Mux1/2  "<t_0 y>"
  Mux1/1 -> [Traffic_Info_20]
  Traffic Object8/1 -> Terminator8/1
  Constant7/1 -> Traffic Object8/1
  Bus Selector7/1 -> Mux1/1  "<t_0 x>"
  Bus Selector10/3 -> Mux13/3  "<r_zyx z>"
  Traffic Object10/2 -> Bus Selector9/1
  Constant11/1 -> Traffic Object11/1
  Bus Selector10/1 -> Mux13/1  "<t_0 x>"
  Traffic Object11/2 -> Bus Selector10/1
  Mux13/1 -> [Traffic_Info_13]
  Bus Selector10/2 -> Mux13/2  "<t_0 y>"
  Mux12/1 -> [Traffic_Info_04]
  Bus Selector9/2 -> Mux12/2  "<t_0 y>"
  Traffic Object11/1 -> Terminator11/1
  Bus Selector9/1 -> Mux12/1  "<t_0 x>"
  Constant9/1 -> Traffic Object10/1
  Traffic Object10/1 -> Terminator10/1
  Bus Selector9/3 -> Mux12/3  "<r_zyx z>"
  Bus Selector14/2 -> Mux15/2  "<t_0 y>"
  Mux15/1 -> [Traffic_Info_05]
  Mux16/1 -> [Traffic_Info_14]
  Traffic Object14/1 -> Terminator14/1
  Bus Selector12/2 -> Mux16/2  "<t_0 y>"
  Traffic Object14/2 -> Bus Selector12/1
  Bus Selector12/1 -> Mux16/1  "<t_0 x>"
  Constant13/1 -> Traffic Object14/1
  Bus Selector12/3 -> Mux16/3  "<r_zyx z>"
  Traffic Object13/2 -> Bus Selector14/1
  Bus Selector14/1 -> Mux15/1  "<t_0 x>"
  Bus Selector14/3 -> Mux15/3  "<r_zyx z>"
  Traffic Object13/1 -> Terminator13/1
  Constant15/1 -> Traffic Object13/1
  Bus Selector17/2 -> Mux18/2  "<t_0 y>"
  Mux18/1 -> [Traffic_Info_06]
  Mux19/1 -> [Traffic_Info_15]
  Traffic Object17/1 -> Terminator17/1
  Bus Selector15/2 -> Mux19/2  "<t_0 y>"
  Traffic Object17/2 -> Bus Selector15/1
  Bus Selector15/1 -> Mux19/1  "<t_0 x>"
  Constant16/1 -> Traffic Object17/1
  Bus Selector15/3 -> Mux19/3  "<r_zyx z>"
  Traffic Object16/2 -> Bus Selector17/1
  Bus Selector17/1 -> Mux18/1  "<t_0 x>"
  Bus Selector17/3 -> Mux18/3  "<r_zyx z>"
  Traffic Object16/1 -> Terminator16/1
  Constant18/1 -> Traffic Object16/1
  Bus Selector20/2 -> Mux21/2  "<t_0 y>"
  Mux21/1 -> [Traffic_Info_07]
  Mux22/1 -> [Traffic_Info_16]
  Traffic Object20/1 -> Terminator20/1
  Bus Selector18/2 -> Mux22/2  "<t_0 y>"
  Traffic Object20/2 -> Bus Selector18/1
  Bus Selector18/1 -> Mux22/1  "<t_0 x>"
  Constant19/1 -> Traffic Object20/1
  Bus Selector18/3 -> Mux22/3  "<r_zyx z>"
  Traffic Object19/2 -> Bus Selector20/1
  Bus Selector20/1 -> Mux21/1  "<t_0 x>"
  Bus Selector20/3 -> Mux21/3  "<r_zyx z>"
  Traffic Object19/1 -> Terminator19/1
  Constant21/1 -> Traffic Object19/1
  Bus Selector23/2 -> Mux24/2  "<t_0 y>"
  Mux24/1 -> [Traffic_Info_08]
  Mux25/1 -> [Traffic_Info_17]
  Traffic Object23/1 -> Terminator23/1
  Bus Selector21/2 -> Mux25/2  "<t_0 y>"
  Traffic Object23/2 -> Bus Selector21/1
  Bus Selector21/1 -> Mux25/1  "<t_0 x>"
  Constant22/1 -> Traffic Object23/1
  Bus Selector21/3 -> Mux25/3  "<r_zyx z>"
  Traffic Object22/2 -> Bus Selector23/1
  Bus Selector23/1 -> Mux24/1  "<t_0 x>"
  Bus Selector23/3 -> Mux24/3  "<r_zyx z>"
  Traffic Object22/1 -> Terminator22/1
  Constant24/1 -> Traffic Object22/1
  Bus Selector26/2 -> Mux27/2  "<t_0 y>"
  Mux27/1 -> [Traffic_Info_09]
  Mux28/1 -> [Traffic_Info_18]
  Traffic Object26/1 -> Terminator26/1
  Bus Selector24/2 -> Mux28/2  "<t_0 y>"
  Traffic Object26/2 -> Bus Selector24/1
  Bus Selector24/1 -> Mux28/1  "<t_0 x>"
  Constant25/1 -> Traffic Object26/1
  Bus Selector24/3 -> Mux28/3  "<r_zyx z>"
  Traffic Object25/2 -> Bus Selector26/1
  Bus Selector26/1 -> Mux27/1  "<t_0 x>"
  Bus Selector26/3 -> Mux27/3  "<r_zyx z>"
  Traffic Object25/1 -> Terminator25/1
  Constant27/1 -> Traffic Object25/1
  [Traffic_Info_01] -> Mux9/1
  [Traffic_Info_02] -> Mux9/2
  [Traffic_Info_03] -> Mux9/3
  [Traffic_Info_04] -> Mux9/4
  [Traffic_Info_05] -> Mux9/5
  [Traffic_Info_06] -> Mux9/6
  [Traffic_Info_07] -> Mux9/7
  [Traffic_Info_08] -> Mux9/8
  [Traffic_Info_09] -> Mux9/9
  [Traffic_Info_10] -> Mux9/10
  [Traffic_Info_11] -> Mux9/11
  [Traffic_Info_12] -> Mux9/12
  [Traffic_Info_13] -> Mux9/13
  [Traffic_Info_14] -> Mux9/14
  [Traffic_Info_15] -> Mux9/15
  [Traffic_Info_16] -> Mux9/16
  [Traffic_Info_17] -> Mux9/17
  [Traffic_Info_18] -> Mux9/18
  [Traffic_Info_19] -> Mux9/19
  [Traffic_Info_20] -> Mux9/20
